simulink model "ProcessNetworkSimulation"  (R2015b)
(part 2 of 21)

  Process_86/RConn6 -- Process_18/LConn36
  Process_86/RConn7 -- Process_19/LConn34
  Process_86/RConn8 -- Process_23/LConn34
  Process_86/RConn9 -- Process_24/LConn29
  Process_86/RConn10 -- Process_25/LConn30
  Process_86/RConn11 -- Process_27/LConn36
  Process_86/RConn12 -- Process_28/LConn26
  Process_86/RConn13 -- Process_32/LConn29
  Process_86/RConn14 -- Process_35/LConn30
  Process_86/RConn15 -- Process_39/LConn31
  Process_86/RConn16 -- Process_40/LConn41
  Process_86/RConn17 -- Process_42/LConn30
  Process_86/RConn18 -- Process_43/LConn33
  Process_86/RConn19 -- Process_45/LConn33
  Process_86/RConn20 -- Process_48/LConn33
  Process_86/RConn21 -- Process_49/LConn32
  Process_86/RConn22 -- Process_50/LConn39
  Process_86/RConn23 -- Process_52/LConn32
  Process_86/RConn24 -- Process_58/LConn38
  Process_86/RConn25 -- Process_61/LConn36
  Process_86/RConn26 -- Process_62/LConn29
  Process_86/RConn27 -- Process_68/LConn36
  Process_86/RConn28 -- Process_72/LConn26
  Process_86/RConn29 -- Process_73/LConn36
  Process_86/RConn30 -- Process_75/LConn38
  Process_86/RConn31 -- Process_79/LConn35
  Process_86/RConn32 -- Process_80/LConn26
  Process_86/RConn33 -- Process_83/LConn39
  Process_86/RConn34 -- Process_84/LConn36
  Process_86/RConn35 -- Process_94/LConn36
  Process_86/RConn36 -- Process_96/LConn35
  Process_86/RConn37 -- Process_99/LConn41
  Process_87/RConn1 -- Process_1/LConn25
  Process_87/RConn2 -- Process_4/LConn34
  Process_87/RConn3 -- Process_7/LConn37
  Process_87/RConn4 -- Process_12/LConn33
  Process_87/RConn5 -- Process_13/LConn37
  Process_87/RConn6 -- Process_23/LConn35
  Process_87/RConn7 -- Process_24/LConn30
  Process_87/RConn8 -- Process_26/LConn36
  Process_87/RConn9 -- Process_28/LConn27
  Process_87/RConn10 -- Process_30/LConn33
  Process_87/RConn11 -- Process_31/LConn24
  Process_87/RConn12 -- Process_34/LConn33
  Process_87/RConn13 -- Process_38/LConn32
  Process_87/RConn14 -- Process_41/LConn44
  Process_87/RConn15 -- Process_43/LConn34
  Process_87/RConn16 -- Process_45/LConn34
  Process_87/RConn17 -- Process_46/LConn36
  Process_87/RConn18 -- Process_47/LConn31
  Process_87/RConn19 -- Process_52/LConn33
  Process_87/RConn20 -- Process_54/LConn35
  Process_87/RConn21 -- Process_56/LConn37
  Process_87/RConn22 -- Process_59/LConn37
  Process_87/RConn23 -- Process_61/LConn37
  Process_87/RConn24 -- Process_65/LConn32
  Process_87/RConn25 -- Process_67/LConn30
  Process_87/RConn26 -- Process_74/LConn29
  Process_87/RConn27 -- Process_76/LConn34
  Process_87/RConn28 -- Process_79/LConn36
  Process_87/RConn29 -- Process_81/LConn31
  Process_87/RConn30 -- Process_84/LConn37
  Process_87/RConn31 -- Process_85/LConn35
  Process_87/RConn32 -- Process_86/LConn32
  Process_87/RConn33 -- Process_90/LConn39
  Process_87/RConn34 -- Process_91/LConn36
  Process_87/RConn35 -- Process_93/LConn34
  Process_87/RConn36 -- Process_94/LConn37
  Process_88/RConn1 -- Process_2/LConn28
  Process_88/RConn2 -- Process_4/LConn35
  Process_88/RConn3 -- Process_9/LConn38
  Process_88/RConn4 -- Process_14/LConn33
  Process_88/RConn5 -- Process_15/LConn36
  Process_88/RConn6 -- Process_20/LConn31
  Process_88/RConn7 -- Process_22/LConn33
  Process_88/RConn8 -- Process_25/LConn31
  Process_88/RConn9 -- Process_32/LConn30
  Process_88/RConn10 -- Process_33/LConn37
  Process_88/RConn11 -- Process_34/LConn34
  Process_88/RConn12 -- Process_35/LConn31
  Process_88/RConn13 -- Process_36/LConn30
  Process_88/RConn14 -- Process_43/LConn35
  Process_88/RConn15 -- Process_49/LConn33
  Process_88/RConn16 -- Process_52/LConn34
  Process_88/RConn17 -- Process_59/LConn38
  Process_88/RConn18 -- Process_60/LConn31
  Process_88/RConn19 -- Process_73/LConn37
  Process_88/RConn20 -- Process_75/LConn39
  Process_88/RConn21 -- Process_76/LConn35
  Process_88/RConn22 -- Process_77/LConn34
  Process_88/RConn23 -- Process_78/LConn25
  Process_88/RConn24 -- Process_79/LConn37
  Process_88/RConn25 -- Process_86/LConn33
  Process_88/RConn26 -- Process_88/LConn27
  Process_88/RConn27 -- Process_91/LConn37
  Process_88/RConn28 -- Process_97/LConn23
  Process_88/RConn29 -- Process_100/LConn30
  Process_89/RConn1 -- Process_1/LConn26
  Process_89/RConn2 -- Process_5/LConn28
  Process_89/RConn3 -- Process_9/LConn39
  Process_89/RConn4 -- Process_10/LConn33
  Process_89/RConn5 -- Process_13/LConn38
  Process_89/RConn6 -- Process_26/LConn37
  Process_89/RConn7 -- Process_27/LConn37
  Process_89/RConn8 -- Process_29/LConn34
  Process_89/RConn9 -- Process_30/LConn34
  Process_89/RConn10 -- Process_31/LConn25
  Process_89/RConn11 -- Process_32/LConn31
  Process_89/RConn12 -- Process_34/LConn35
  Process_89/RConn13 -- Process_35/LConn32
  Process_89/RConn14 -- Process_40/LConn42
  Process_89/RConn15 -- Process_43/LConn36
  Process_89/RConn16 -- Process_44/LConn38
  Process_89/RConn17 -- Process_46/LConn37
  Process_89/RConn18 -- Process_51/LConn36
  Process_89/RConn19 -- Process_54/LConn36
  Process_89/RConn20 -- Process_55/LConn43
  Process_89/RConn21 -- Process_61/LConn38
  Process_89/RConn22 -- Process_63/LConn38
  Process_89/RConn23 -- Process_69/LConn34
  Process_89/RConn24 -- Process_74/LConn30
  Process_89/RConn25 -- Process_75/LConn40
  Process_89/RConn26 -- Process_77/LConn35
  Process_89/RConn27 -- Process_79/LConn38
  Process_89/RConn28 -- Process_80/LConn27
  Process_89/RConn29 -- Process_81/LConn32
  Process_89/RConn30 -- Process_82/LConn36
  Process_89/RConn31 -- Process_83/LConn40
  Process_89/RConn32 -- Process_84/LConn38
  Process_89/RConn33 -- Process_85/LConn36
  Process_89/RConn34 -- Process_87/LConn31
  Process_89/RConn35 -- Process_90/LConn40
  Process_89/RConn36 -- Process_93/LConn35
  Process_89/RConn37 -- Process_96/LConn36
  Process_89/RConn38 -- Process_98/LConn36
  Process_89/RConn39 -- Process_99/LConn42
  Process_90/RConn1 -- Process_1/LConn27
  Process_90/RConn2 -- Process_2/LConn29
  Process_90/RConn3 -- Process_5/LConn29
  Process_90/RConn4 -- Process_6/LConn41
  Process_90/RConn5 -- Process_8/LConn30
  Process_90/RConn6 -- Process_14/LConn34
  Process_90/RConn7 -- Process_16/LConn36
  Process_90/RConn8 -- Process_17/LConn38
  Process_90/RConn9 -- Process_18/LConn37
  Process_90/RConn10 -- Process_24/LConn31
  Process_90/RConn11 -- Process_25/LConn32
  Process_90/RConn12 -- Process_26/LConn38
  Process_90/RConn13 -- Process_29/LConn35
  Process_90/RConn14 -- Process_31/LConn26
  Process_90/RConn15 -- Process_35/LConn33
  Process_90/RConn16 -- Process_36/LConn31
  Process_90/RConn17 -- Process_37/LConn32
  Process_90/RConn18 -- Process_38/LConn33
  Process_90/RConn19 -- Process_39/LConn32
  Process_90/RConn20 -- Process_40/LConn43
  Process_90/RConn21 -- Process_42/LConn31
  Process_90/RConn22 -- Process_45/LConn35
  Process_90/RConn23 -- Process_48/LConn34
  Process_90/RConn24 -- Process_52/LConn35
  Process_90/RConn25 -- Process_57/LConn26
  Process_90/RConn26 -- Process_61/LConn39
  Process_90/RConn27 -- Process_66/LConn35
  Process_90/RConn28 -- Process_67/LConn31
  Process_90/RConn29 -- Process_72/LConn27
  Process_90/RConn30 -- Process_73/LConn38
  Process_90/RConn31 -- Process_75/LConn41
  Process_90/RConn32 -- Process_76/LConn36
  Process_90/RConn33 -- Process_80/LConn28
  Process_90/RConn34 -- Process_86/LConn34
  Process_90/RConn35 -- Process_88/LConn28
  Process_90/RConn36 -- Process_91/LConn38
  Process_90/RConn37 -- Process_92/LConn34
  Process_90/RConn38 -- Process_93/LConn36
  Process_90/RConn39 -- Process_95/LConn25
  Process_91/RConn1 -- Process_10/LConn34
  Process_91/RConn2 -- Process_11/LConn41
  Process_91/RConn3 -- Process_13/LConn39
  Process_91/RConn4 -- Process_15/LConn37
  Process_91/RConn5 -- Process_20/LConn32
  Process_91/RConn6 -- Process_24/LConn32
  Process_91/RConn7 -- Process_27/LConn38
  Process_91/RConn8 -- Process_30/LConn35
  Process_91/RConn9 -- Process_31/LConn27
  Process_91/RConn10 -- Process_32/LConn32
  Process_91/RConn11 -- Process_35/LConn34
  Process_91/RConn12 -- Process_40/LConn44
  Process_91/RConn13 -- Process_44/LConn39
  Process_91/RConn14 -- Process_45/LConn36
  Process_91/RConn15 -- Process_48/LConn35
  Process_91/RConn16 -- Process_53/LConn30
  Process_91/RConn17 -- Process_58/LConn39
  Process_91/RConn18 -- Process_59/LConn39
  Process_91/RConn19 -- Process_61/LConn40
  Process_91/RConn20 -- Process_62/LConn30
  Process_91/RConn21 -- Process_63/LConn39
  Process_91/RConn22 -- Process_64/LConn30
  Process_91/RConn23 -- Process_65/LConn33
  Process_91/RConn24 -- Process_66/LConn36
  Process_91/RConn25 -- Process_67/LConn32
  Process_91/RConn26 -- Process_68/LConn37
  Process_91/RConn27 -- Process_70/LConn29
  Process_91/RConn28 -- Process_72/LConn28
  Process_91/RConn29 -- Process_73/LConn39
  Process_91/RConn30 -- Process_74/LConn31
  Process_91/RConn31 -- Process_75/LConn42
  Process_91/RConn32 -- Process_76/LConn37
  Process_91/RConn33 -- Process_78/LConn26
  Process_91/RConn34 -- Process_80/LConn29
  Process_91/RConn35 -- Process_85/LConn37
  Process_91/RConn36 -- Process_86/LConn35
  Process_91/RConn37 -- Process_87/LConn32
  Process_91/RConn38 -- Process_89/LConn42
  Process_91/RConn39 -- Process_90/LConn41
  Process_91/RConn40 -- Process_92/LConn35
  Process_91/RConn41 -- Process_94/LConn38
  Process_91/RConn42 -- Process_95/LConn26
  Process_91/RConn43 -- Process_96/LConn37
  Process_91/RConn44 -- Process_99/LConn43
  Process_92/RConn1 -- Process_1/LConn28
  Process_92/RConn2 -- Process_2/LConn30
  Process_92/RConn3 -- Process_10/LConn35
  Process_92/RConn4 -- Process_14/LConn35
  Process_92/RConn5 -- Process_16/LConn37
  Process_92/RConn6 -- Process_19/LConn35
  Process_92/RConn7 -- Process_20/LConn33
  Process_92/RConn8 -- Process_22/LConn34
  Process_92/RConn9 -- Process_25/LConn33
  Process_92/RConn10 -- Process_27/LConn39
  Process_92/RConn11 -- Process_30/LConn36
  Process_92/RConn12 -- Process_33/LConn38
  Process_92/RConn13 -- Process_36/LConn32
  Process_92/RConn14 -- Process_39/LConn33
  Process_92/RConn15 -- Process_40/LConn45
  Process_92/RConn16 -- Process_45/LConn37
  Process_92/RConn17 -- Process_47/LConn32
  Process_92/RConn18 -- Process_49/LConn34
  Process_92/RConn19 -- Process_53/LConn31
  Process_92/RConn20 -- Process_54/LConn37
  Process_92/RConn21 -- Process_58/LConn40
  Process_92/RConn22 -- Process_61/LConn41
  Process_92/RConn23 -- Process_62/LConn31
  Process_92/RConn24 -- Process_64/LConn31
  Process_92/RConn25 -- Process_66/LConn37
  Process_92/RConn26 -- Process_69/LConn35
  Process_92/RConn27 -- Process_77/LConn36
  Process_92/RConn28 -- Process_80/LConn30
  Process_92/RConn29 -- Process_81/LConn33
  Process_92/RConn30 -- Process_82/LConn37
  Process_92/RConn31 -- Process_90/LConn42
  Process_92/RConn32 -- Process_91/LConn39
  Process_92/RConn33 -- Process_97/LConn24
  Process_92/RConn34 -- Process_98/LConn37
  Process_92/RConn35 -- Process_99/LConn44
  Process_93/RConn1 -- Process_1/LConn29
  Process_93/RConn2 -- Process_2/LConn31
  Process_93/RConn3 -- Process_3/LConn30
  Process_93/RConn4 -- Process_4/LConn36
  Process_93/RConn5 -- Process_5/LConn30
  Process_93/RConn6 -- Process_8/LConn31
  Process_93/RConn7 -- Process_9/LConn40
  Process_93/RConn8 -- Process_10/LConn36
  Process_93/RConn9 -- Process_13/LConn40
  Process_93/RConn10 -- Process_14/LConn36
  Process_93/RConn11 -- Process_23/LConn36
  Process_93/RConn12 -- Process_30/LConn37
  Process_93/RConn13 -- Process_31/LConn28
  Process_93/RConn14 -- Process_32/LConn33
  Process_93/RConn15 -- Process_37/LConn33
  Process_93/RConn16 -- Process_43/LConn37
  Process_93/RConn17 -- Process_47/LConn33
  Process_93/RConn18 -- Process_50/LConn40
  Process_93/RConn19 -- Process_52/LConn36
  Process_93/RConn20 -- Process_55/LConn44
  Process_93/RConn21 -- Process_56/LConn38
  Process_93/RConn22 -- Process_57/LConn27
  Process_93/RConn23 -- Process_58/LConn41
  Process_93/RConn24 -- Process_61/LConn42
  Process_93/RConn25 -- Process_63/LConn40
  Process_93/RConn26 -- Process_64/LConn32
  Process_93/RConn27 -- Process_66/LConn38
  Process_93/RConn28 -- Process_67/LConn33
  Process_93/RConn29 -- Process_68/LConn38
  Process_93/RConn30 -- Process_70/LConn30
  Process_93/RConn31 -- Process_74/LConn32
  Process_93/RConn32 -- Process_77/LConn37
  Process_93/RConn33 -- Process_79/LConn39
  Process_93/RConn34 -- Process_82/LConn38
  Process_93/RConn35 -- Process_83/LConn41
  Process_93/RConn36 -- Process_85/LConn38
  Process_93/RConn37 -- Process_87/LConn33
  Process_93/RConn38 -- Process_94/LConn39
  Process_93/RConn39 -- Process_98/LConn38
  Process_94/RConn1 -- Process_1/LConn30
  Process_94/RConn2 -- Process_4/LConn37
  Process_94/RConn3 -- Process_6/LConn42
  Process_94/RConn4 -- Process_8/LConn32
  Process_94/RConn5 -- Process_9/LConn41
  Process_94/RConn6 -- Process_12/LConn34
  Process_94/RConn7 -- Process_20/LConn34
  Process_94/RConn8 -- Process_21/LConn29
  Process_94/RConn9 -- Process_22/LConn35
  Process_94/RConn10 -- Process_24/LConn33
  Process_94/RConn11 -- Process_25/LConn34
  Process_94/RConn12 -- Process_27/LConn40
  Process_94/RConn13 -- Process_28/LConn28
  Process_94/RConn14 -- Process_31/LConn29
  Process_94/RConn15 -- Process_34/LConn36
  Process_94/RConn16 -- Process_35/LConn35
  Process_94/RConn17 -- Process_36/LConn33
  Process_94/RConn18 -- Process_41/LConn45
  Process_94/RConn19 -- Process_45/LConn38
  Process_94/RConn20 -- Process_47/LConn34
  Process_94/RConn21 -- Process_48/LConn36
  Process_94/RConn22 -- Process_51/LConn37
  Process_94/RConn23 -- Process_53/LConn32
  Process_94/RConn24 -- Process_54/LConn38
  Process_94/RConn25 -- Process_59/LConn40
  Process_94/RConn26 -- Process_65/LConn34
  Process_94/RConn27 -- Process_66/LConn39
  Process_94/RConn28 -- Process_68/LConn39
  Process_94/RConn29 -- Process_70/LConn31
  Process_94/RConn30 -- Process_74/LConn33
  Process_94/RConn31 -- Process_77/LConn38
  Process_94/RConn32 -- Process_79/LConn40
  Process_94/RConn33 -- Process_81/LConn34
  Process_94/RConn34 -- Process_82/LConn39
  Process_94/RConn35 -- Process_83/LConn42
  Process_94/RConn36 -- Process_84/LConn39
  Process_94/RConn37 -- Process_86/LConn36
  Process_94/RConn38 -- Process_88/LConn29
  Process_94/RConn39 -- Process_90/LConn43
  Process_94/RConn40 -- Process_92/LConn36
  Process_94/RConn41 -- Process_93/LConn37
  Process_94/RConn42 -- Process_94/LConn40
  Process_94/RConn43 -- Process_100/LConn31
  Process_95/RConn1 -- Process_4/LConn38
  Process_95/RConn2 -- Process_9/LConn42
  Process_95/RConn3 -- Process_10/LConn37
  Process_95/RConn4 -- Process_13/LConn41
  Process_95/RConn5 -- Process_14/LConn37
  Process_95/RConn6 -- Process_22/LConn36
  Process_95/RConn7 -- Process_26/LConn39
  Process_95/RConn8 -- Process_30/LConn38
  Process_95/RConn9 -- Process_31/LConn30
  Process_95/RConn10 -- Process_35/LConn36
  Process_95/RConn11 -- Process_38/LConn34
  Process_95/RConn12 -- Process_39/LConn34
  Process_95/RConn13 -- Process_40/LConn46
  Process_95/RConn14 -- Process_43/LConn38
  Process_95/RConn15 -- Process_44/LConn40
  Process_95/RConn16 -- Process_45/LConn39
  Process_95/RConn17 -- Process_46/LConn38
  Process_95/RConn18 -- Process_47/LConn35
  Process_95/RConn19 -- Process_48/LConn37
  Process_95/RConn20 -- Process_49/LConn35
  Process_95/RConn21 -- Process_50/LConn41
  Process_95/RConn22 -- Process_57/LConn28
  Process_95/RConn23 -- Process_58/LConn42
  Process_95/RConn24 -- Process_61/LConn43
  Process_95/RConn25 -- Process_64/LConn33
  Process_95/RConn26 -- Process_65/LConn35
  Process_95/RConn27 -- Process_68/LConn40
  Process_95/RConn28 -- Process_71/LConn35
  Process_95/RConn29 -- Process_72/LConn29
  Process_95/RConn30 -- Process_74/LConn34
  Process_95/RConn31 -- Process_78/LConn27
  Process_95/RConn32 -- Process_81/LConn35
  Process_95/RConn33 -- Process_84/LConn40
  Process_95/RConn34 -- Process_93/LConn38
  Process_96/RConn1 -- Process_1/LConn31
  Process_96/RConn2 -- Process_3/LConn31
  Process_96/RConn3 -- Process_4/LConn39
  Process_96/RConn4 -- Process_8/LConn33
  Process_96/RConn5 -- Process_10/LConn38
  Process_96/RConn6 -- Process_13/LConn42
  Process_96/RConn7 -- Process_15/LConn38
  Process_96/RConn8 -- Process_20/LConn35
  Process_96/RConn9 -- Process_23/LConn37
  Process_96/RConn10 -- Process_25/LConn35
  Process_96/RConn11 -- Process_26/LConn40
  Process_96/RConn12 -- Process_28/LConn29
  Process_96/RConn13 -- Process_29/LConn36
  Process_96/RConn14 -- Process_36/LConn34
  Process_96/RConn15 -- Process_38/LConn35
  Process_96/RConn16 -- Process_41/LConn46
  Process_96/RConn17 -- Process_45/LConn40
  Process_96/RConn18 -- Process_46/LConn39
  Process_96/RConn19 -- Process_49/LConn36
  Process_96/RConn20 -- Process_50/LConn42
  Process_96/RConn21 -- Process_51/LConn38
  Process_96/RConn22 -- Process_53/LConn33
  Process_96/RConn23 -- Process_55/LConn45
  Process_96/RConn24 -- Process_57/LConn29
  Process_96/RConn25 -- Process_60/LConn32
  Process_96/RConn26 -- Process_63/LConn41
  Process_96/RConn27 -- Process_68/LConn41
  Process_96/RConn28 -- Process_70/LConn32
  Process_96/RConn29 -- Process_71/LConn36
  Process_96/RConn30 -- Process_74/LConn35
  Process_96/RConn31 -- Process_75/LConn43
  Process_96/RConn32 -- Process_76/LConn38
  Process_96/RConn33 -- Process_78/LConn28
  Process_96/RConn34 -- Process_79/LConn41
  Process_96/RConn35 -- Process_80/LConn31
  Process_96/RConn36 -- Process_83/LConn43
  Process_96/RConn37 -- Process_84/LConn41
  Process_96/RConn38 -- Process_86/LConn37
  Process_96/RConn39 -- Process_88/LConn30
  Process_96/RConn40 -- Process_89/LConn43
  Process_96/RConn41 -- Process_90/LConn44
  Process_96/RConn42 -- Process_91/LConn40
  Process_96/RConn43 -- Process_93/LConn39
  Process_96/RConn44 -- Process_96/LConn38
  Process_96/RConn45 -- Process_97/LConn25
  Process_96/RConn46 -- Process_98/LConn39
  Process_97/RConn1 -- Process_1/LConn32
  Process_97/RConn2 -- Process_2/LConn32
  Process_97/RConn3 -- Process_4/LConn40
  Process_97/RConn4 -- Process_5/LConn31
  Process_97/RConn5 -- Process_6/LConn43
  Process_97/RConn6 -- Process_7/LConn38
  Process_97/RConn7 -- Process_8/LConn34
  Process_97/RConn8 -- Process_10/LConn39
  Process_97/RConn9 -- Process_13/LConn43
  Process_97/RConn10 -- Process_21/LConn30
  Process_97/RConn11 -- Process_24/LConn34
  Process_97/RConn12 -- Process_26/LConn41
  Process_97/RConn13 -- Process_33/LConn39
  Process_97/RConn14 -- Process_36/LConn35
  Process_97/RConn15 -- Process_39/LConn35
  Process_97/RConn16 -- Process_47/LConn36
  Process_97/RConn17 -- Process_48/LConn38
  Process_97/RConn18 -- Process_52/LConn37
  Process_97/RConn19 -- Process_54/LConn39
  Process_97/RConn20 -- Process_59/LConn41
  Process_97/RConn21 -- Process_61/LConn44
  Process_97/RConn22 -- Process_68/LConn42
  Process_97/RConn23 -- Process_72/LConn30
  Process_97/RConn24 -- Process_77/LConn39
  Process_97/RConn25 -- Process_84/LConn42
  Process_97/RConn26 -- Process_89/LConn44
  Process_97/RConn27 -- Process_90/LConn45
  Process_97/RConn28 -- Process_95/LConn27
  Process_97/RConn29 -- Process_98/LConn40
  Process_98/RConn1 -- Process_4/LConn41
  Process_98/RConn2 -- Process_5/LConn32
  Process_98/RConn3 -- Process_7/LConn39
  Process_98/RConn4 -- Process_10/LConn40
  Process_98/RConn5 -- Process_12/LConn35
  Process_98/RConn6 -- Process_14/LConn38
  Process_98/RConn7 -- Process_16/LConn38
  Process_98/RConn8 -- Process_18/LConn38
  Process_98/RConn9 -- Process_22/LConn37
  Process_98/RConn10 -- Process_24/LConn35
  Process_98/RConn11 -- Process_35/LConn37
  Process_98/RConn12 -- Process_38/LConn36
  Process_98/RConn13 -- Process_39/LConn36
  Process_98/RConn14 -- Process_40/LConn47
  Process_98/RConn15 -- Process_42/LConn32
  Process_98/RConn16 -- Process_46/LConn40
  Process_98/RConn17 -- Process_50/LConn43
  Process_98/RConn18 -- Process_57/LConn30
  Process_98/RConn19 -- Process_59/LConn42
  Process_98/RConn20 -- Process_60/LConn33
  Process_98/RConn21 -- Process_62/LConn32
  Process_98/RConn22 -- Process_64/LConn34
  Process_98/RConn23 -- Process_65/LConn36
  Process_98/RConn24 -- Process_68/LConn43
  Process_98/RConn25 -- Process_69/LConn36
  Process_98/RConn26 -- Process_72/LConn31
  Process_98/RConn27 -- Process_73/LConn40
  Process_98/RConn28 -- Process_80/LConn32
  Process_98/RConn29 -- Process_81/LConn36
  Process_98/RConn30 -- Process_82/LConn40
  Process_98/RConn31 -- Process_83/LConn44
  Process_98/RConn32 -- Process_85/LConn39
  Process_98/RConn33 -- Process_88/LConn31
  Process_98/RConn34 -- Process_89/LConn45
  Process_98/RConn35 -- Process_96/LConn39
  Process_98/RConn36 -- Process_97/LConn26
  Process_98/RConn37 -- Process_100/LConn32
  Process_99/RConn1 -- Process_3/LConn32
  Process_99/RConn2 -- Process_13/LConn44
  Process_99/RConn3 -- Process_17/LConn39
  Process_99/RConn4 -- Process_21/LConn31
  Process_99/RConn5 -- Process_22/LConn38
  Process_99/RConn6 -- Process_25/LConn36
  Process_99/RConn7 -- Process_29/LConn37
  Process_99/RConn8 -- Process_32/LConn34
  Process_99/RConn9 -- Process_34/LConn37
  Process_99/RConn10 -- Process_36/LConn36
  Process_99/RConn11 -- Process_38/LConn37
  Process_99/RConn12 -- Process_43/LConn39
  Process_99/RConn13 -- Process_48/LConn39
  Process_99/RConn14 -- Process_52/LConn38
  Process_99/RConn15 -- Process_57/LConn31
  Process_99/RConn16 -- Process_59/LConn43
  Process_99/RConn17 -- Process_61/LConn45
  Process_99/RConn18 -- Process_62/LConn33
  Process_99/RConn19 -- Process_63/LConn42
  Process_99/RConn20 -- Process_64/LConn35
  Process_99/RConn21 -- Process_65/LConn37
  Process_99/RConn22 -- Process_66/LConn40
  Process_99/RConn23 -- Process_70/LConn33
  Process_99/RConn24 -- Process_71/LConn37
  Process_99/RConn25 -- Process_74/LConn36
  Process_99/RConn26 -- Process_77/LConn40
  Process_99/RConn27 -- Process_79/LConn42
  Process_99/RConn28 -- Process_81/LConn37
  Process_99/RConn29 -- Process_83/LConn45
  Process_99/RConn30 -- Process_85/LConn40
  Process_99/RConn31 -- Process_87/LConn34
  Process_99/RConn32 -- Process_88/LConn32
  Process_99/RConn33 -- Process_89/LConn46
  Process_99/RConn34 -- Process_90/LConn46
  Process_99/RConn35 -- Process_96/LConn40
  Process_99/RConn36 -- Process_97/LConn27
  Process_99/RConn37 -- Process_98/LConn41
  Process_99/RConn38 -- Process_99/LConn45
  Process_99/RConn39 -- Process_100/LConn33
  Process_100/RConn1 -- Process_7/LConn40
  Process_100/RConn2 -- Process_12/LConn36
  Process_100/RConn3 -- Process_15/LConn39
  Process_100/RConn4 -- Process_20/LConn36
  Process_100/RConn5 -- Process_21/LConn32
  Process_100/RConn6 -- Process_24/LConn36
  Process_100/RConn7 -- Process_25/LConn37
  Process_100/RConn8 -- Process_26/LConn42
  Process_100/RConn9 -- Process_30/LConn39
  Process_100/RConn10 -- Process_38/LConn38
  Process_100/RConn11 -- Process_41/LConn47
  Process_100/RConn12 -- Process_42/LConn33
  Process_100/RConn13 -- Process_47/LConn37
  Process_100/RConn14 -- Process_48/LConn40
  Process_100/RConn15 -- Process_53/LConn34
  Process_100/RConn16 -- Process_55/LConn46
  Process_100/RConn17 -- Process_57/LConn32
  Process_100/RConn18 -- Process_59/LConn44
  Process_100/RConn19 -- Process_60/LConn34
  Process_100/RConn20 -- Process_62/LConn34
  Process_100/RConn21 -- Process_63/LConn43
  Process_100/RConn22 -- Process_73/LConn41
  Process_100/RConn23 -- Process_81/LConn38
  Process_100/RConn24 -- Process_86/LConn38
  Process_100/RConn25 -- Process_87/LConn35
  Process_100/RConn26 -- Process_93/LConn40
  Process_100/RConn27 -- Process_96/LConn41
  Process_100/RConn28 -- Process_97/LConn28
  Process_100/RConn29 -- Process_100/LConn34
  Arrival_Process/RConn1 -- Process_1/LConn33
  Arrival_Process/RConn2 -- Process_2/LConn33
  Arrival_Process/RConn3 -- Process_3/LConn33
  Arrival_Process/RConn4 -- Process_4/LConn42
  Arrival_Process/RConn5 -- Process_5/LConn33
  Arrival_Process/RConn6 -- Process_6/LConn44
  Arrival_Process/RConn7 -- Process_7/LConn41
  Arrival_Process/RConn8 -- Process_8/LConn35
  Arrival_Process/RConn9 -- Process_9/LConn43
  Arrival_Process/RConn10 -- Process_10/LConn41
  Arrival_Process/RConn11 -- Process_11/LConn42
  Arrival_Process/RConn12 -- Process_12/LConn37
  Arrival_Process/RConn13 -- Process_13/LConn45
  Arrival_Process/RConn14 -- Process_14/LConn39
  Arrival_Process/RConn15 -- Process_15/LConn40
  Arrival_Process/RConn16 -- Process_16/LConn39
  Arrival_Process/RConn17 -- Process_17/LConn40
  Arrival_Process/RConn18 -- Process_18/LConn39
  Arrival_Process/RConn19 -- Process_19/LConn36
  Arrival_Process/RConn20 -- Process_20/LConn37
  Arrival_Process/RConn21 -- Process_21/LConn33
  Arrival_Process/RConn22 -- Process_22/LConn39
  Arrival_Process/RConn23 -- Process_23/LConn38
  Arrival_Process/RConn24 -- Process_24/LConn37
  Arrival_Process/RConn25 -- Process_25/LConn38
  Arrival_Process/RConn26 -- Process_26/LConn43
  Arrival_Process/RConn27 -- Process_27/LConn41
  Arrival_Process/RConn28 -- Process_28/LConn30
  Arrival_Process/RConn29 -- Process_29/LConn38
  Arrival_Process/RConn30 -- Process_30/LConn40
  Arrival_Process/RConn31 -- Process_31/LConn31
  Arrival_Process/RConn32 -- Process_32/LConn35
  Arrival_Process/RConn33 -- Process_33/LConn40
  Arrival_Process/RConn34 -- Process_34/LConn38
  Arrival_Process/RConn35 -- Process_35/LConn38
  Arrival_Process/RConn36 -- Process_36/LConn37
  Arrival_Process/RConn37 -- Process_37/LConn34
  Arrival_Process/RConn38 -- Process_38/LConn39
  Arrival_Process/RConn39 -- Process_39/LConn37
  Arrival_Process/RConn40 -- Process_40/LConn48
  Arrival_Process/RConn41 -- Process_41/LConn48
  Arrival_Process/RConn42 -- Process_42/LConn34
  Arrival_Process/RConn43 -- Process_43/LConn40
  Arrival_Process/RConn44 -- Process_44/LConn41
  Arrival_Process/RConn45 -- Process_45/LConn41
  Arrival_Process/RConn46 -- Process_46/LConn41
  Arrival_Process/RConn47 -- Process_47/LConn38
  Arrival_Process/RConn48 -- Process_48/LConn41
  Arrival_Process/RConn49 -- Process_49/LConn37
  Arrival_Process/RConn50 -- Process_50/LConn44
  Arrival_Process/RConn51 -- Process_51/LConn39
  Arrival_Process/RConn52 -- Process_52/LConn39
  Arrival_Process/RConn53 -- Process_53/LConn35
  Arrival_Process/RConn54 -- Process_54/LConn40
  Arrival_Process/RConn55 -- Process_55/LConn47
  Arrival_Process/RConn56 -- Process_56/LConn39
  Arrival_Process/RConn57 -- Process_57/LConn33
  Arrival_Process/RConn58 -- Process_58/LConn43
  Arrival_Process/RConn59 -- Process_59/LConn45
  Arrival_Process/RConn60 -- Process_60/LConn35
  Arrival_Process/RConn61 -- Process_61/LConn46
  Arrival_Process/RConn62 -- Process_62/LConn35
  Arrival_Process/RConn63 -- Process_63/LConn44
  Arrival_Process/RConn64 -- Process_64/LConn36
  Arrival_Process/RConn65 -- Process_65/LConn38
  Arrival_Process/RConn66 -- Process_66/LConn41
  Arrival_Process/RConn67 -- Process_67/LConn34
  Arrival_Process/RConn68 -- Process_68/LConn44
  Arrival_Process/RConn69 -- Process_69/LConn37
  Arrival_Process/RConn70 -- Process_70/LConn34
  Arrival_Process/RConn71 -- Process_71/LConn38
  Arrival_Process/RConn72 -- Process_72/LConn32
  Arrival_Process/RConn73 -- Process_73/LConn42
  Arrival_Process/RConn74 -- Process_74/LConn37
  Arrival_Process/RConn75 -- Process_75/LConn44
  Arrival_Process/RConn76 -- Process_76/LConn39
  Arrival_Process/RConn77 -- Process_77/LConn41
  Arrival_Process/RConn78 -- Process_78/LConn29
  Arrival_Process/RConn79 -- Process_79/LConn43
  Arrival_Process/RConn80 -- Process_80/LConn33
  Arrival_Process/RConn81 -- Process_81/LConn39
  Arrival_Process/RConn82 -- Process_82/LConn41
  Arrival_Process/RConn83 -- Process_83/LConn46
  Arrival_Process/RConn84 -- Process_84/LConn43
  Arrival_Process/RConn85 -- Process_85/LConn41
  Arrival_Process/RConn86 -- Process_86/LConn39
  Arrival_Process/RConn87 -- Process_87/LConn36
  Arrival_Process/RConn88 -- Process_88/LConn33
  Arrival_Process/RConn89 -- Process_89/LConn47
  Arrival_Process/RConn90 -- Process_90/LConn47
  Arrival_Process/RConn91 -- Process_91/LConn41
  Arrival_Process/RConn92 -- Process_92/LConn37
  Arrival_Process/RConn93 -- Process_93/LConn41
  Arrival_Process/RConn94 -- Process_94/LConn41
  Arrival_Process/RConn95 -- Process_95/LConn28
  Arrival_Process/RConn96 -- Process_96/LConn42
  Arrival_Process/RConn97 -- Process_97/LConn29
  Arrival_Process/RConn98 -- Process_98/LConn42
  Arrival_Process/RConn99 -- Process_99/LConn46
  Arrival_Process/RConn100 -- Process_100/LConn35
  Process_1/RConn37 -- Departure_Process/LConn1
  Process_2/RConn32 -- Departure_Process/LConn2
  Process_3/RConn31 -- Departure_Process/LConn3
  Process_4/RConn37 -- Departure_Process/LConn4
  Process_6/RConn39 -- Departure_Process/LConn5
  Process_7/RConn42 -- Departure_Process/LConn6
  Process_8/RConn34 -- Departure_Process/LConn7
  Process_9/RConn43 -- Departure_Process/LConn8
  Process_10/RConn41 -- Departure_Process/LConn9
  Process_12/RConn41 -- Departure_Process/LConn10
  Process_13/RConn42 -- Departure_Process/LConn11
  Process_14/RConn40 -- Departure_Process/LConn12
  Process_17/RConn33 -- Departure_Process/LConn13
  Process_21/RConn34 -- Departure_Process/LConn14
  Process_23/RConn36 -- Departure_Process/LConn15
  Process_25/RConn41 -- Departure_Process/LConn16
  Process_26/RConn40 -- Departure_Process/LConn17
  Process_27/RConn43 -- Departure_Process/LConn18
  Process_28/RConn29 -- Departure_Process/LConn19
  Process_31/RConn28 -- Departure_Process/LConn20
  Process_34/RConn40 -- Departure_Process/LConn21
  Process_35/RConn38 -- Departure_Process/LConn22
  Process_40/RConn45 -- Departure_Process/LConn23
  Process_43/RConn42 -- Departure_Process/LConn24
  Process_46/RConn41 -- Departure_Process/LConn25
  Process_47/RConn34 -- Departure_Process/LConn26
  Process_48/RConn37 -- Departure_Process/LConn27
  Process_51/RConn38 -- Departure_Process/LConn28
  Process_53/RConn39 -- Departure_Process/LConn29
  Process_55/RConn46 -- Departure_Process/LConn30
  Process_57/RConn32 -- Departure_Process/LConn31
  Process_58/RConn43 -- Departure_Process/LConn32
  Process_60/RConn41 -- Departure_Process/LConn33
  Process_62/RConn41 -- Departure_Process/LConn34
  Process_63/RConn42 -- Departure_Process/LConn35
  Process_64/RConn36 -- Departure_Process/LConn36
  Process_66/RConn42 -- Departure_Process/LConn37
  Process_67/RConn35 -- Departure_Process/LConn38
  Process_69/RConn41 -- Departure_Process/LConn39
  Process_70/RConn37 -- Departure_Process/LConn40
  Process_73/RConn44 -- Departure_Process/LConn41
  Process_74/RConn35 -- Departure_Process/LConn42
  Process_75/RConn50 -- Departure_Process/LConn43
  Process_76/RConn38 -- Departure_Process/LConn44
  Process_77/RConn38 -- Departure_Process/LConn45
  Process_79/RConn39 -- Departure_Process/LConn46
  Process_80/RConn41 -- Departure_Process/LConn47
  Process_81/RConn38 -- Departure_Process/LConn48
  Process_83/RConn45 -- Departure_Process/LConn49
  Process_85/RConn38 -- Departure_Process/LConn50
  Process_86/RConn38 -- Departure_Process/LConn51
  Process_87/RConn37 -- Departure_Process/LConn52
  Process_89/RConn40 -- Departure_Process/LConn53
  Process_90/RConn40 -- Departure_Process/LConn54
  Process_91/RConn45 -- Departure_Process/LConn55
  Process_92/RConn36 -- Departure_Process/LConn56
  Process_93/RConn40 -- Departure_Process/LConn57
  Process_94/RConn44 -- Departure_Process/LConn58
  Process_96/RConn47 -- Departure_Process/LConn59
  Process_97/RConn30 -- Departure_Process/LConn60
  Process_99/RConn40 -- Departure_Process/LConn61
  Process_100/RConn30 -- Departure_Process/LConn62
